simulink model "Three_Phase_Inverter_Model"  (R2021a)
settings: Solver=VariableStepAuto  StartTime=0.0  StopTime=1/60  RelTol=1e-3
libraries: spsIGBTLib x6, spsSeriesRLCBranchLib x3, spsDCVoltageSourceLib x1, spsMultimeterLib x1, spspowerguiLib x1
settings Model: Creator=Pichau  LastModifiedBy=Pichau

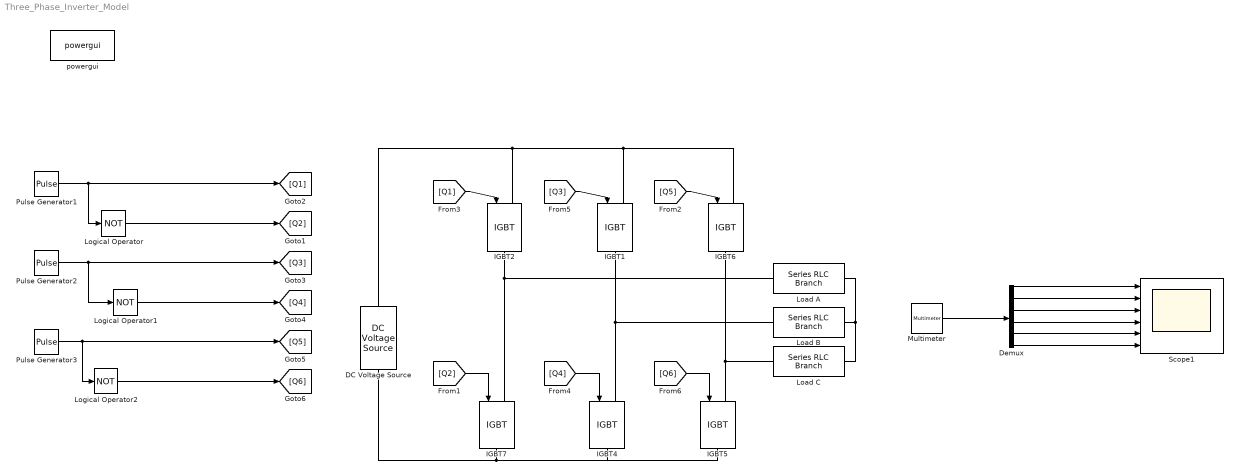
== system Three_Phase_Inverter_Model ==
  DC Voltage Source : spsDCVoltageSourceLib/DC Voltage Source  Amplitude=100  Measurements=None
  Demux : Demux  Outputs=6
  IGBT{1..2,4..7} (6 alike) : spsIGBTLib/IGBT  Ron=0.001  Lon=0  Vf=1  Tf=1e-6  Tt=2e-6  IC=0  Rs=1e5  Cs=inf  Measurements=off
  Load A : spsSeriesRLCBranchLib/Series RLC Branch  LConnTagsString=__new0  RConnTagsString=__new0  BranchType=R  Resistance=10  Inductance=1e-3  SetiL0=off  InitialCurrent=0  Capacitance=1e-6  Setx0=off  InitialVoltage=0  Measurements=Branch voltage and current
  Load B : spsSeriesRLCBranchLib/Series RLC Branch  LConnTagsString=__new0  RConnTagsString=__new0  BranchType=R  Resistance=10  Inductance=1e-3  SetiL0=off  InitialCurrent=0  Capacitance=1e-6  Setx0=off  InitialVoltage=0  Measurements=Branch voltage and current
  Load C : spsSeriesRLCBranchLib/Series RLC Branch  LConnTagsString=__new0  RConnTagsString=__new0  BranchType=R  Resistance=10  Inductance=1e-3  SetiL0=off  InitialCurrent=0  Capacitance=1e-6  Setx0=off  InitialVoltage=0  Measurements=Branch voltage and current
  Logical Operator : Logic  Operator=NOT  AllPortsSameDT=off  OutDataTypeStr=boolean
  Logical Operator1 : Logic  Operator=NOT  AllPortsSameDT=off  OutDataTypeStr=boolean
  Logical Operator2 : Logic  Operator=NOT  AllPortsSameDT=off  OutDataTypeStr=boolean
  Multimeter : spsMultimeterLib/Multimeter  PhasorSimulation=off  OutputType=Complex  sel=[1 2 3 4 5 6]  L=6  Gain=[1 1 1 1 1 1]  yselected={'Ub: Load A','Ub: Load B','Ub: Load C','Ib: Load A','Ib: Load B','Ib: Load C'};  PSBOutputType=1  PSBequivalent=0  AxesSetting=[0,0.1,-100,100]  Display=0  SavedBlockNames=-11
  Pulse Generator1 : DiscretePulseGenerator  PulseType=Time based  Period=1/60  PulseWidth=50
  Pulse Generator2 : DiscretePulseGenerator  PulseType=Time based  Period=1/60  PulseWidth=50  PhaseDelay=-240/360*(1/60)
  Pulse Generator3 : DiscretePulseGenerator  PulseType=Time based  Period=1/60  PulseWidth=50  PhaseDelay=-120/360*(1/60)
  Scope1 : Scope  NumInputPorts=6
  powergui : spspowerguiLib/powergui  Priority=1  SimulationMode=Continuous  SampleTime=50e-6  frequency=60  Iterations=50  frequencyindice=0  Pbase=100e6  ErrMax=1e-4  UnitsV=kV  UnitsW=MW  buscounter=0  FunctionMessages=off  echomessages=off  EnableUseOfTLC=off  CurrentSourceSwitches=off  DisableSnubberDevices=off  DisableRonSwitches=off  DisableVfSwitches=off  DisplayEquations=off  AutomaticDiscreteSolvers=off  SolverType=Tustin/Backward Euler (TBE)  Interpol=off  ExternalGateDelay=off  methode=off  Ts=100  x0status=blocks  SPID=on  SwTol=0  HookPort=off  NonlinearTolerance=1e-4  nMaxIteration=100  ContinueOnMaxIteration=off  RestoreLinks=warning  ResistiveCurrentMeasurement=off  Frange=[0:2:500]  Ylog=off  Xlog=on  ShowGrid=off  save=off  variable=ZData  structure=0  ZoomFFT=off  StartTime=0.0  cycles=1  DisplayStyle=1  fundamental=60  FreqAxis=off  MaxFrequency=1000  frequencyindicesteady=1  RmsSteady=1  display=off
  wires:
  Pulse Generator1/1 -> Logical Operator/1, [Q1]
  Logical Operator/1 -> [Q2]
  Logical Operator1/1 -> [Q4]
  Pulse Generator2/1 -> [Q3], Logical Operator1/1
  Pulse Generator3/1 -> [Q5], Logical Operator2/1
  Logical Operator2/1 -> [Q6]
  [Q1] -> IGBT2/1
  [Q2] -> IGBT7/1
  [Q3] -> IGBT1/1
  [Q4] -> IGBT4/1
  [Q5] -> IGBT6/1
  [Q6] -> IGBT5/1
  Demux/5 -> Scope1/5
  Demux/6 -> Scope1/6
  Demux/3 -> Scope1/3
  Demux/2 -> Scope1/2
  Demux/1 -> Scope1/1
  Multimeter/1 -> Demux/1
  Demux/4 -> Scope1/4
  connections:
  DC Voltage Source/RConn1 -- IGBT6/LConn1 -- IGBT1/LConn1 -- IGBT2/LConn1
  IGBT7/LConn1 -- Load A/LConn1 -- IGBT2/RConn1
  IGBT4/LConn1 -- IGBT1/RConn1 -- Load B/LConn1
  IGBT5/LConn1 -- IGBT6/RConn1 -- Load C/LConn1
  DC Voltage Source/LConn1 -- IGBT5/RConn1 -- IGBT4/RConn1 -- IGBT7/RConn1
  Load B/RConn1 -- Load A/RConn1 -- Load C/RConn1
